simulink model "ab"  (Simulink 7.3)
settings: Solver=ode45  StartTime=0.0  StopTime=1000  FixedStep=0.01  RelTol=1e-9  AbsTol=1e-12
settings Model: Creator=ec1099  LastModifiedBy=ec1099
settings DataIOCC: LimitDataPoints=off  SaveOutput=off  SignalLogging=off  SaveTime=off
settings OptimizationCC: InlineParams=on  InitFltsAndDblsToZero=on  SimCompilerOptimization=On
settings DebuggingCC: SolverPrmCheckMsg=none

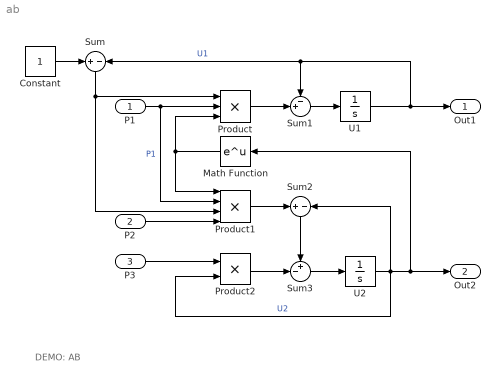
== system ab ==
  note: DEMO: AB
  P1 : Inport  OutDataType=sfix(16)  OutScaling=2^0
  P2 : Inport  Port=2  OutDataType=sfix(16)  OutScaling=2^0
  P3 : Inport  Port=3  OutDataType=sfix(16)  OutScaling=2^0
  Constant : Constant  OutDataType=sfix(16)  OutScaling=2^0
  Math Function : Math  OutDataType=sfix(16)  OutScaling=2^0  SaturateOnIntegerOverflow=on
  Product : Product  Inputs=3  OutDataType=sfix(16)  OutScaling=2^0  RndMeth=Zero
  Product1 : Product  Inputs=4  OutDataType=sfix(16)  OutScaling=2^0  RndMeth=Zero
  Product2 : Product  OutDataType=sfix(16)  OutScaling=2^0  RndMeth=Zero
  Sum : Sum  Inputs=+-  OutDataType=sfix(16)  OutScaling=2^0
  Sum1 : Sum  Inputs=-+|  OutDataType=sfix(16)  OutScaling=2^0
  Sum2 : Sum  Inputs=+-  OutDataType=sfix(16)  OutScaling=2^0
  Sum3 : Sum  Inputs=+-|  OutDataType=sfix(16)  OutScaling=2^0
  U1 : Integrator
  U2 : Integrator
  Out1 : Outport  OutDataType=sfix(16)  OutScaling=2^0
  Out2 : Outport  Port=2  OutDataType=sfix(16)  OutScaling=2^0
  wires:
  U1/1 -> Sum/2, Sum1/1, Out1/1  "U1"
  Constant/1 -> Sum/1
  U2/1 -> Sum2/2, Product2/2, Math Function/1, Out2/1  "U2"
  Math Function/1 -> Product/3, Product1/1
  P1/1 -> Product/2, Product1/2  "P1"
  Sum/1 -> Product/1, Product1/3
  Sum1/1 -> U1/1
  Product/1 -> Sum1/2
  P2/1 -> Product1/4
  Product1/1 -> Sum2/1
  P3/1 -> Product2/1
  Product2/1 -> Sum3/2
  Sum2/1 -> Sum3/1
  Sum3/1 -> U2/1
